simulink subsystem "HO_CAN"  (R2019b)
settings: Solver=VariableStepAuto  StartTime=0.0  StopTime=10.0  RelTol=1e-3
libraries: canmsglib x8, c280xlib x7, FunctionCallDivider x4
settings Model: Creator=Nick  LastModifiedBy=Nick

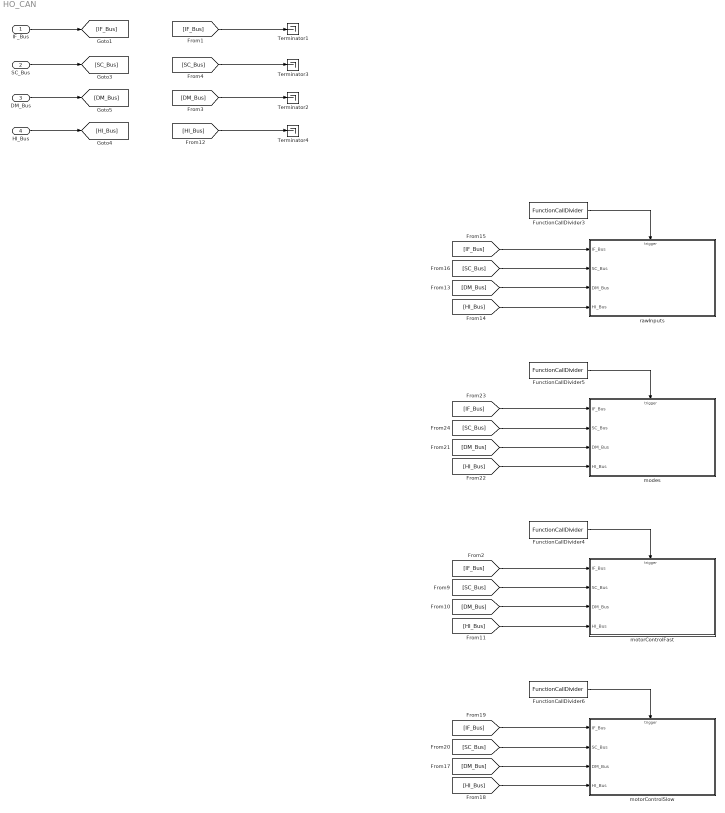
== system HO_CAN ==
  IF_Bus : Inport
  SC_Bus : Inport  Port=2
  DM_Bus : Inport  Port=3
  HI_Bus : Inport  Port=4
  FunctionCallDivider3 : FunctionCallDivider/Algroithms/FunctionCallDivider  counts=10
  FunctionCallDivider4 : FunctionCallDivider/Algroithms/FunctionCallDivider  counts=1
  FunctionCallDivider5 : FunctionCallDivider/Algroithms/FunctionCallDivider  counts=100
  FunctionCallDivider6 : FunctionCallDivider/Algroithms/FunctionCallDivider  counts=10
  Terminator{1..4} (4 alike) : Terminator
  modes : Subsystem  TreatAsAtomicUnit=on
  motorControlFast : Subsystem  TreatAsAtomicUnit=on
  motorControlSlow : Subsystem  TreatAsAtomicUnit=on
  rawInputs : Subsystem  TreatAsAtomicUnit=on
  wires:
  FunctionCallDivider4/1 -> motorControlFast/Trigger
  [DM_Bus] -> motorControlFast/3(DM_Bus)
  [IF_Bus] -> motorControlSlow/1(IF_Bus)
  [SC_Bus] -> motorControlFast/2(SC_Bus)
  FunctionCallDivider6/1 -> motorControlSlow/Trigger
  [HI_Bus] -> motorControlFast/4(HI_Bus)
  [DM_Bus] -> motorControlSlow/3(DM_Bus)
  [HI_Bus] -> motorControlSlow/4(HI_Bus)
  [SC_Bus] -> motorControlSlow/2(SC_Bus)
  [IF_Bus] -> motorControlFast/1(IF_Bus)
  [SC_Bus] -> modes/2(SC_Bus)
  [HI_Bus] -> modes/4(HI_Bus)
  [IF_Bus] -> modes/1(IF_Bus)
  [DM_Bus] -> modes/3(DM_Bus)
  FunctionCallDivider5/1 -> modes/Trigger
  IF_Bus/1 -> [IF_Bus]
  [HI_Bus] -> Terminator4/1
  HI_Bus/1 -> [HI_Bus]
  SC_Bus/1 -> [SC_Bus]
  DM_Bus/1 -> [DM_Bus]
  [SC_Bus] -> Terminator3/1
  [DM_Bus] -> Terminator2/1
  [IF_Bus] -> Terminator1/1
  [HI_Bus] -> rawInputs/4(HI_Bus)
  [IF_Bus] -> rawInputs/1(IF_Bus)
  FunctionCallDivider3/1 -> rawInputs/Trigger
  [DM_Bus] -> rawInputs/3(DM_Bus)
  [SC_Bus] -> rawInputs/2(SC_Bus)

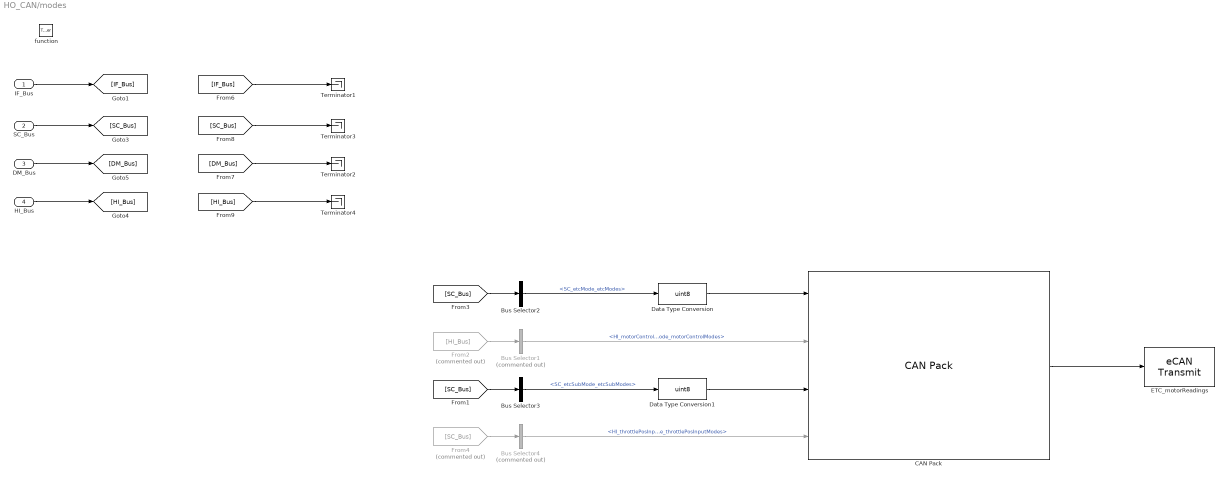
== system HO_CAN/modes ==
  IF_Bus : Inport
  SC_Bus : Inport  Port=2
  DM_Bus : Inport  Port=3
  HI_Bus : Inport  Port=4
  function : TriggerPort  TriggerType=function-call  VariantControl=Variant
  Bus Selector1 : BusSelector  Commented=on  OutputSignals=VectorBoxBus.HI_motorControlMode_motorControlModes
  Bus Selector2 : BusSelector  OutputSignals=modeControlBus.SC_etcMode_etcModes
  Bus Selector3 : BusSelector  OutputSignals=modeControlBus.SC_etcSubMode_etcSubModes
  Bus Selector4 : BusSelector  Commented=on  OutputSignals=VectorBoxBus.HI_throttlePosInputMode_throttlePosInputModes
  CAN Pack : canmsglib/CAN Pack  CANdbFile=C:\Git\ETC-Development\DBCs\F28379D_etc_benchTest_CAN2.dbc  MsgList=ETC_modes  MsgName=ETC_modes  MsgIDType=Standard (11-bit identifier)  MsgIdentifier=110  MsgLength=4  Remote=off  ApplyMinMax=off  BusOutput=off  SignalInfo={'ETC_mode','0','8','LE','unsigned','Standard','0','1','0','0','255';'ETC_motorControlMode','16','8','LE','unsigned','Standard','0','1','0','0','255';'ETC_subMode','8','8','LE','unsigned','Standard','0','1','0','0','255';'ETC_throttlePosInputMode','24','8','LE','unsigned','Standard','0','1','0','0','255'}
      settings: SourceProductName=Vehicle Network Toolbox  SourceProductBaseCode=VN  DataFormat=CANdb specified signals
  Data Type Conversion : DataTypeConversion  OutDataTypeStr=uint8
  Data Type Conversion1 : DataTypeConversion  OutDataTypeStr=uint8
  ETC_motorReadings : c280xlib/eCAN Transmit  chipFamily=C280x  useModule=eCAN_A  mailboxNo=6  messageID=0  messageType=Standard (11-bit identifier)  enableBlockingMode=off  postInterrupt=off  interruptLine=0
      settings: SourceProductName=Embedded Coder Support Package for Texas Instruments C2000 Processors  SourceProductBaseCode=TIC2000
  From2 : From  Commented=on  GotoTag=HI_Bus
  From4 : From  Commented=on  GotoTag=SC_Bus
  Terminator{1..4} (4 alike) : Terminator
  wires:
  From4/1 -> Bus Selector4/1
  Bus Selector4/1 -> CAN Pack/4  "<HI_throttlePosInputMode_throttlePosInputModes>"
  [SC_Bus] -> Bus Selector3/1
  Bus Selector3/1 -> Data Type Conversion1/1  "<SC_etcSubMode_etcSubModes>"
  IF_Bus/1 -> [IF_Bus]
  [HI_Bus] -> Terminator4/1
  HI_Bus/1 -> [HI_Bus]
  SC_Bus/1 -> [SC_Bus]
  DM_Bus/1 -> [DM_Bus]
  [SC_Bus] -> Terminator3/1
  [DM_Bus] -> Terminator2/1
  [IF_Bus] -> Terminator1/1
  Bus Selector1/1 -> CAN Pack/2  "<HI_motorControlMode_motorControlModes>"
  Bus Selector2/1 -> Data Type Conversion/1  "<SC_etcMode_etcModes>"
  From2/1 -> Bus Selector1/1
  [SC_Bus] -> Bus Selector2/1
  CAN Pack/1 -> ETC_motorReadings/1
  Data Type Conversion/1 -> CAN Pack/1
  Data Type Conversion1/1 -> CAN Pack/3

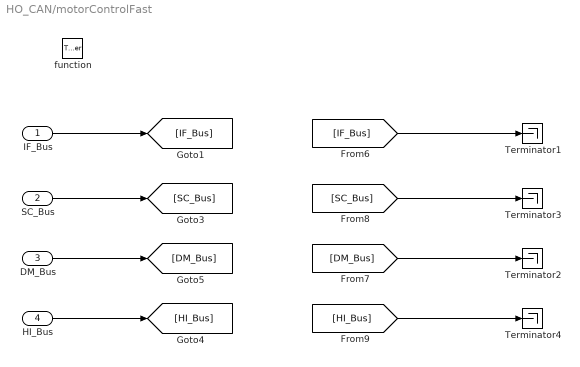
== system HO_CAN/motorControlFast ==
  IF_Bus : Inport
  SC_Bus : Inport  Port=2
  DM_Bus : Inport  Port=3
  HI_Bus : Inport  Port=4
  function : TriggerPort  TriggerType=function-call  VariantControl=Variant
  Terminator{1..4} (4 alike) : Terminator
  wires:
  IF_Bus/1 -> [IF_Bus]
  [HI_Bus] -> Terminator4/1
  HI_Bus/1 -> [HI_Bus]
  SC_Bus/1 -> [SC_Bus]
  DM_Bus/1 -> [DM_Bus]
  [SC_Bus] -> Terminator3/1
  [DM_Bus] -> Terminator2/1
  [IF_Bus] -> Terminator1/1

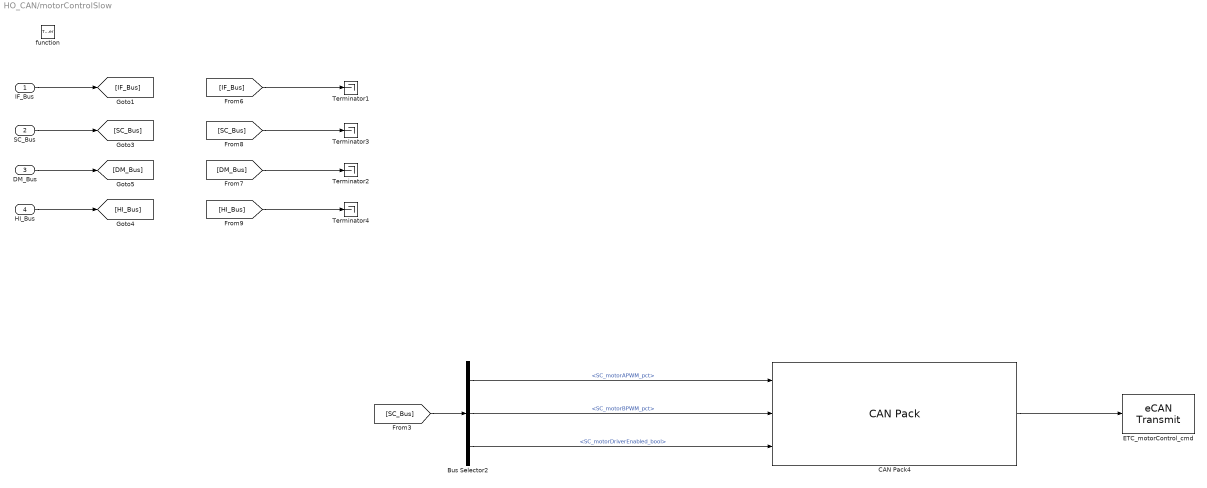
== system HO_CAN/motorControlSlow ==
  IF_Bus : Inport
  SC_Bus : Inport  Port=2
  DM_Bus : Inport  Port=3
  HI_Bus : Inport  Port=4
  function : TriggerPort  TriggerType=function-call  VariantControl=Variant
  Bus Selector2 : BusSelector  OutputSignals=motorControlBus.SC_motorAPWM_pct,motorControlBus.SC_motorBPWM_pct,motorControlBus.SC_motorDriverEnabled_bool
  CAN Pack4 : canmsglib/CAN Pack  CANdbFile=C:\Git\ETC-Development\DBCs\F28379D_etc_benchTest_CAN2.dbc  MsgList=ETC_motorControl_cmd  MsgName=ETC_motorControl_cmd  MsgIDType=Standard (11-bit identifier)  MsgIdentifier=111  MsgLength=8  Remote=off  ApplyMinMax=off  BusOutput=off  SignalInfo={'ETC_motorAPWM','0','8','LE','unsigned','Standard','0','1','0','0','255';'ETC_motorBPWM','8','8','LE','unsigned','Standard','0','1','0','0','255';'ETC_motorDriverEnabled','16','1','LE','unsigned','Standard','0','1','0','0','1'}
      settings: SourceProductName=Vehicle Network Toolbox  SourceProductBaseCode=VN  DataFormat=CANdb specified signals
  ETC_motorControl_cmd : c280xlib/eCAN Transmit  chipFamily=C280x  useModule=eCAN_B  mailboxNo=7  messageID=0  messageType=Standard (11-bit identifier)  enableBlockingMode=off  postInterrupt=off  interruptLine=0
      settings: SourceProductName=Embedded Coder Support Package for Texas Instruments C2000 Processors  SourceProductBaseCode=TIC2000
  Terminator{1..4} (4 alike) : Terminator
  wires:
  Bus Selector2/3 -> CAN Pack4/3  "<SC_motorDriverEnabled_bool>"
  Bus Selector2/2 -> CAN Pack4/2  "<SC_motorBPWM_pct>"
  Bus Selector2/1 -> CAN Pack4/1  "<SC_motorAPWM_pct>"
  [SC_Bus] -> Bus Selector2/1
  IF_Bus/1 -> [IF_Bus]
  [HI_Bus] -> Terminator4/1
  HI_Bus/1 -> [HI_Bus]
  SC_Bus/1 -> [SC_Bus]
  DM_Bus/1 -> [DM_Bus]
  [SC_Bus] -> Terminator3/1
  [DM_Bus] -> Terminator2/1
  [IF_Bus] -> Terminator1/1
  CAN Pack4/1 -> ETC_motorControl_cmd/1

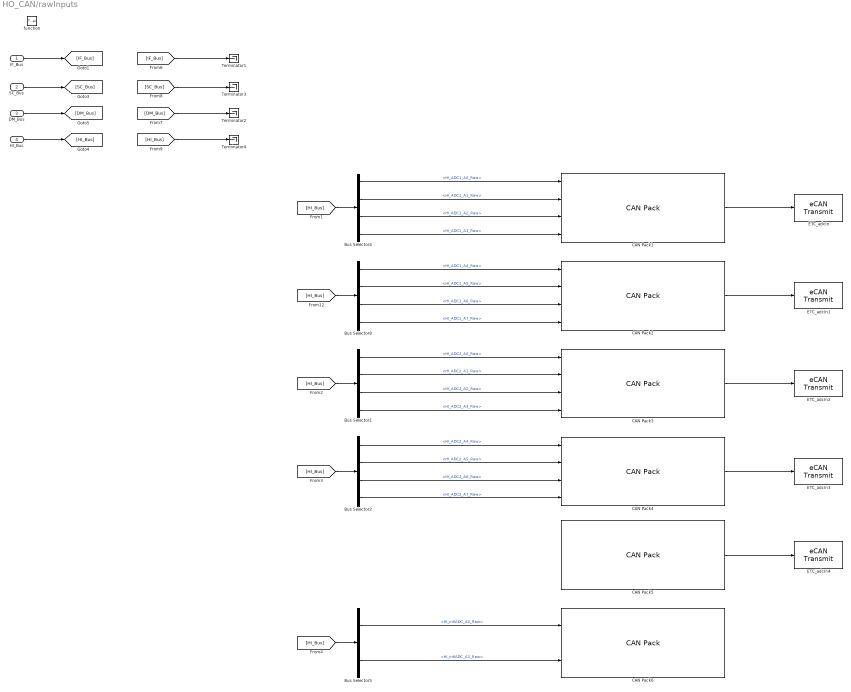
== system HO_CAN/rawInputs ==
  IF_Bus : Inport
  SC_Bus : Inport  Port=2
  DM_Bus : Inport  Port=3
  HI_Bus : Inport  Port=4
  function : TriggerPort  TriggerType=function-call  VariantControl=Variant
  Bus Selector1 : BusSelector  OutputSignals=SPIBus.ADC2Bus.HI_ADC2_A0_Raw,SPIBus.ADC2Bus.HI_ADC2_A1_Raw,SPIBus.ADC2Bus.HI_ADC2_A2_Raw,SPIBus.ADC2Bus.HI_ADC2_A3_Raw
  Bus Selector2 : BusSelector  OutputSignals=SPIBus.ADC2Bus.HI_ADC2_A4_Raw,SPIBus.ADC2Bus.HI_ADC2_A5_Raw,SPIBus.ADC2Bus.HI_ADC2_A6_Raw,SPIBus.ADC2Bus.HI_ADC2_A7_Raw
  Bus Selector4 : BusSelector  OutputSignals=SPIBus.ADC1Bus.HI_ADC1_A0_Raw,SPIBus.ADC1Bus.HI_ADC1_A1_Raw,SPIBus.ADC1Bus.HI_ADC1_A2_Raw,SPIBus.ADC1Bus.HI_ADC1_A3_Raw
  Bus Selector5 : BusSelector  OutputSignals=AnalogBus.HI_intlADC_A2_Raw,AnalogBus.HI_intlADC_A3_Raw
  Bus Selector8 : BusSelector  OutputSignals=SPIBus.ADC1Bus.HI_ADC1_A4_Raw,SPIBus.ADC1Bus.HI_ADC1_A5_Raw,SPIBus.ADC1Bus.HI_ADC1_A6_Raw,SPIBus.ADC1Bus.HI_ADC1_A7_Raw
  CAN Pack1 : canmsglib/CAN Pack  CANdbFile=C:\Git\ETC-Development\DBCs\F28379D_etc_benchTest_CAN2.dbc  MsgList=ETC_adcRaw1  MsgName=ETC_adcRaw1  MsgIDType=Standard (11-bit identifier)  MsgIdentifier=135  MsgLength=8  Remote=off  ApplyMinMax=off  BusOutput=off  SignalInfo={'ETC_extADC1_A0_Raw','0','16','LE','unsigned','Standard','0','1','0','-Inf','Inf';'ETC_extADC1_A1_Raw','16','16','LE','unsigned','Standard','0','1','0','-Inf','Inf';'ETC_extADC1_A2_Raw','32','16','LE','unsigned','Standard','0','1','0','-Inf','Inf';'ETC_extADC1_A3_Raw','48','16','LE','unsigned','Standard','0','1','0','-Inf','Inf'}
      settings: SourceProductName=Vehicle Network Toolbox  SourceProductBaseCode=VN  DataFormat=CANdb specified signals
  CAN Pack2 : canmsglib/CAN Pack  CANdbFile=C:\Git\ETC-Development\DBCs\F28379D_etc_benchTest_CAN2.dbc  MsgList=ETC_adcRaw2  MsgName=ETC_adcRaw2  MsgIDType=Standard (11-bit identifier)  MsgIdentifier=136  MsgLength=8  Remote=off  ApplyMinMax=off  BusOutput=off  SignalInfo={'ETC_extADC1_A4_Raw','0','16','LE','unsigned','Standard','0','1','0','-Inf','Inf';'ETC_extADC1_A5_Raw','16','16','LE','unsigned','Standard','0','1','0','-Inf','Inf';'ETC_extADC1_A6_Raw','32','16','LE','unsigned','Standard','0','1','0','-Inf','Inf';'ETC_extADC1_A7_Raw','48','16','LE','unsigned','Standard','0','1','0','-Inf','Inf'}
      settings: SourceProductName=Vehicle Network Toolbox  SourceProductBaseCode=VN  DataFormat=CANdb specified signals
  CAN Pack3 : canmsglib/CAN Pack  CANdbFile=C:\Git\ETC-Development\DBCs\F28379D_etc_benchTest_CAN2.dbc  MsgList=ETC_adcRaw3  MsgName=ETC_adcRaw3  MsgIDType=Standard (11-bit identifier)  MsgIdentifier=137  MsgLength=8  Remote=off  ApplyMinMax=off  BusOutput=off  SignalInfo={'ETC_extADC2_A0_Raw','0','16','LE','unsigned','Standard','0','1','0','-Inf','Inf';'ETC_extADC2_A1_Raw','16','16','LE','unsigned','Standard','0','1','0','-Inf','Inf';'ETC_extADC2_A2_Raw','32','16','LE','unsigned','Standard','0','1','0','-Inf','Inf';'ETC_extADC2_A3_Raw','48','16','LE','unsigned','Standard','0','1','0','-Inf','Inf'}
      settings: SourceProductName=Vehicle Network Toolbox  SourceProductBaseCode=VN  DataFormat=CANdb specified signals
  CAN Pack4 : canmsglib/CAN Pack  CANdbFile=C:\Git\ETC-Development\DBCs\F28379D_etc_benchTest_CAN2.dbc  MsgList=ETC_adcRaw4  MsgName=ETC_adcRaw4  MsgIDType=Standard (11-bit identifier)  MsgIdentifier=138  MsgLength=8  Remote=off  ApplyMinMax=off  BusOutput=off  SignalInfo={'ETC_extADC2_A4_Raw','0','16','LE','unsigned','Standard','0','1','0','-Inf','Inf';'ETC_extADC2_A5_Raw','16','16','LE','unsigned','Standard','0','1','0','-Inf','Inf';'ETC_extADC2_A6_Raw','32','16','LE','unsigned','Standard','0','1','0','-Inf','Inf';'ETC_extADC2_A7_Raw','48','16','LE','unsigned','Standard','0','1','0','-Inf','Inf'}
      settings: SourceProductName=Vehicle Network Toolbox  SourceProductBaseCode=VN  DataFormat=CANdb specified signals
  CAN Pack5 : canmsglib/CAN Pack  CANdbFile=C:\Git\ETC-Development\DBCs\F28379D_etc_benchTest_CAN2.dbc  MsgList=ETC_adcRaw5  MsgName=ETC_adcRaw5  MsgIDType=Standard (11-bit identifier)  MsgIdentifier=139  MsgLength=8  Remote=off  ApplyMinMax=off  BusOutput=off  SignalInfo={'ETC_intlADC_B2_Raw','0','16','LE','unsigned','Standard','0','1','0','-Inf','Inf';'ETC_intlADC_B3_Raw','16','16','LE','unsigned','Standard','0','1','0','-Inf','Inf';'ETC_intlADC_C2_Raw','32','16','LE','unsigned','Standard','0','1','0','-Inf','Inf';'ETC_intlADC_C3_Raw','48','16','LE','unsigned','Standard','0','1','0','-Inf','Inf'}
      settings: SourceProductName=Vehicle Network Toolbox  SourceProductBaseCode=VN  DataFormat=CANdb specified signals
  CAN Pack6 : canmsglib/CAN Pack  CANdbFile=C:\Git\ETC-Development\DBCs\F28379D_etc_benchTest_CAN2.dbc  MsgList=ETC_adcRaw6  MsgName=ETC_adcRaw6  MsgIDType=Standard (11-bit identifier)  MsgIdentifier=140  MsgLength=4  Remote=off  ApplyMinMax=off  BusOutput=off  SignalInfo={'ETC_intlADC_A2_Raw','0','16','LE','unsigned','Standard','0','1','0','-Inf','Inf';'ETC_intlADC_A3_Raw','16','16','LE','unsigned','Standard','0','1','0','-Inf','Inf'}
      settings: SourceProductName=Vehicle Network Toolbox  SourceProductBaseCode=VN  DataFormat=CANdb specified signals
  ETC_adcIn : c280xlib/eCAN Transmit  chipFamily=C280x  useModule=eCAN_B  mailboxNo=0  messageID=0  messageType=Standard (11-bit identifier)  enableBlockingMode=off  postInterrupt=off  interruptLine=0
      settings: SourceProductName=Embedded Coder Support Package for Texas Instruments C2000 Processors  SourceProductBaseCode=TIC2000
  ETC_adcIn1 : c280xlib/eCAN Transmit  chipFamily=C280x  useModule=eCAN_B  mailboxNo=1  messageID=0  messageType=Standard (11-bit identifier)  enableBlockingMode=off  postInterrupt=off  interruptLine=0
      settings: SourceProductName=Embedded Coder Support Package for Texas Instruments C2000 Processors  SourceProductBaseCode=TIC2000
  ETC_adcIn2 : c280xlib/eCAN Transmit  chipFamily=C280x  useModule=eCAN_B  mailboxNo=2  messageID=0  messageType=Standard (11-bit identifier)  enableBlockingMode=off  postInterrupt=off  interruptLine=0
      settings: SourceProductName=Embedded Coder Support Package for Texas Instruments C2000 Processors  SourceProductBaseCode=TIC2000
  ETC_adcIn3 : c280xlib/eCAN Transmit  chipFamily=C280x  useModule=eCAN_B  mailboxNo=3  messageID=0  messageType=Standard (11-bit identifier)  enableBlockingMode=off  postInterrupt=off  interruptLine=0
      settings: SourceProductName=Embedded Coder Support Package for Texas Instruments C2000 Processors  SourceProductBaseCode=TIC2000
  ETC_adcIn4 : c280xlib/eCAN Transmit  chipFamily=C280x  useModule=eCAN_B  mailboxNo=4  messageID=0  messageType=Standard (11-bit identifier)  enableBlockingMode=off  postInterrupt=off  interruptLine=0
      settings: SourceProductName=Embedded Coder Support Package for Texas Instruments C2000 Processors  SourceProductBaseCode=TIC2000
  Terminator{1..4} (4 alike) : Terminator
  wires:
  Bus Selector2/2 -> CAN Pack4/2  "<HI_ADC2_A5_Raw>"
  Bus Selector1/4 -> CAN Pack3/4  "<HI_ADC2_A3_Raw>"
  Bus Selector1/3 -> CAN Pack3/3  "<HI_ADC2_A2_Raw>"
  Bus Selector1/2 -> CAN Pack3/2  "<HI_ADC2_A1_Raw>"
  [HI_Bus] -> Bus Selector1/1
  CAN Pack4/1 -> ETC_adcIn3/1
  [HI_Bus] -> Bus Selector2/1
  CAN Pack3/1 -> ETC_adcIn2/1
  Bus Selector1/1 -> CAN Pack3/1  "<HI_ADC2_A0_Raw>"
  Bus Selector2/1 -> CAN Pack4/1  "<HI_ADC2_A4_Raw>"
  Bus Selector2/3 -> CAN Pack4/3  "<HI_ADC2_A6_Raw>"
  Bus Selector2/4 -> CAN Pack4/4  "<HI_ADC2_A7_Raw>"
  Bus Selector8/4 -> CAN Pack2/4  "<HI_ADC1_A7_Raw>"
  Bus Selector8/3 -> CAN Pack2/3  "<HI_ADC1_A6_Raw>"
  Bus Selector8/2 -> CAN Pack2/2  "<HI_ADC1_A5_Raw>"
  Bus Selector8/1 -> CAN Pack2/1  "<HI_ADC1_A4_Raw>"
  Bus Selector4/1 -> CAN Pack1/1  "<HI_ADC1_A0_Raw>"
  [HI_Bus] -> Bus Selector4/1
  CAN Pack1/1 -> ETC_adcIn/1
  CAN Pack2/1 -> ETC_adcIn1/1
  [HI_Bus] -> Bus Selector8/1
  Bus Selector4/4 -> CAN Pack1/4  "<HI_ADC1_A3_Raw>"
  Bus Selector4/3 -> CAN Pack1/3  "<HI_ADC1_A2_Raw>"
  Bus Selector4/2 -> CAN Pack1/2  "<HI_ADC1_A1_Raw>"
  [IF_Bus] -> Terminator1/1
  [DM_Bus] -> Terminator2/1
  [SC_Bus] -> Terminator3/1
  DM_Bus/1 -> [DM_Bus]
  SC_Bus/1 -> [SC_Bus]
  HI_Bus/1 -> [HI_Bus]
  [HI_Bus] -> Terminator4/1
  IF_Bus/1 -> [IF_Bus]
  Bus Selector5/1 -> CAN Pack6/1  "<HI_intlADC_A2_Raw>"
  Bus Selector5/2 -> CAN Pack6/2  "<HI_intlADC_A3_Raw>"
  CAN Pack5/1 -> ETC_adcIn4/1
  [HI_Bus] -> Bus Selector5/1
